simulink library "marine_gnc"  (Simulink 7.4)
settings: Solver=ode45  SolverMode=SingleTasking  StartTime=0.0  StopTime=10.0  RelTol=1e-3
undefined symbols (not defined in the file or in its folder): CN_data, CX_data, CY_data, D, G, K_supply, kt2ms, M, MA, magnitude, marine, Models, MRB, order, pathlength, RAO_Amp, RAO_Dir, RAO_Freq, RAO_Phase, RAO_Vel, RAO_yaw_back, RAO_yaw_quant, RAO_yaw_quantization_flag, rho_a, Semi, sub, T_supply, table, Tanker, vessel, Vessels
libraries: marine_gnc x64, simulink x39, cybersealib x1
(part 3 of 6)

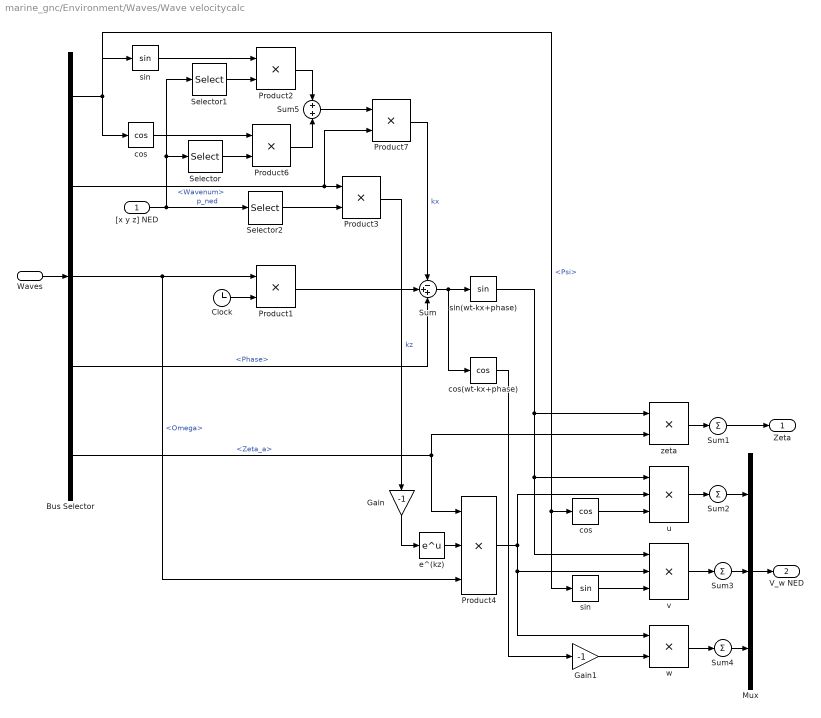
== system marine_gnc/Environment/Waves/Wave velocitycalc ==
  "[x y z] NED" : Inport  OutDataType=sfix(16)  OutScaling=2^0
  Waves : Inport  Port=2  OutDataType=sfix(16)  OutScaling=2^0
  Bus Selector : BusSelector  OutputSignals=Psi,Wavenum,Omega,Phase,Zeta_a
  Clock : Clock
      settings: Decimation=10
  Gain : Gain  Gain=-1  ParameterDataType=sfix(16)  ParameterScaling=2^0  OutDataType=sfix(16)  OutScaling=2^0  SaturateOnIntegerOverflow=on  OutDataTypeStr=Inherit: Same as input  ParamDataTypeStr=Inherit: Same as input
  Gain1 : Gain  Gain=-1  ParameterDataType=sfix(16)  ParameterScaling=2^0  OutDataType=sfix(16)  OutScaling=2^0  SaturateOnIntegerOverflow=on  OutDataTypeStr=Inherit: Same as input  ParamDataTypeStr=Inherit: Same as input
  Mux : Mux  Inputs=3
  Product{1..3,6..7} (5 alike) : Product  Inputs=**  OutDataType=sfix(16)  OutScaling=2^0  SaturateOnIntegerOverflow=on  OutDataTypeStr=Inherit: Same as first input
  Product4 : Product  Inputs=3  OutDataType=sfix(16)  OutScaling=2^0  SaturateOnIntegerOverflow=on  OutDataTypeStr=Inherit: Same as first input
  Selector : Selector  InputPortWidth=3  IndexOptions=Index vector (dialog)  Indices=1  OutputSizes=1
  Selector1 : Selector  InputPortWidth=3  IndexOptions=Index vector (dialog)  Indices=2  OutputSizes=1
  Selector2 : Selector  InputPortWidth=3  IndexOptions=Index vector (dialog)  Indices=3  OutputSizes=1
  Sum : Sum  Inputs=-++  OutDataType=sfix(16)  OutScaling=2^0  SaturateOnIntegerOverflow=on
  Sum{1..4} (4 alike) : Sum  Inputs=1  OutDataType=sfix(16)  OutScaling=2^0  SaturateOnIntegerOverflow=on
  Sum5 : Sum  OutDataType=sfix(16)  OutScaling=2^0  SaturateOnIntegerOverflow=on
  cos : Trigonometry  Operator=cos
  "cos " : Trigonometry  Operator=cos
  cos(wt-kx+phase) : Trigonometry  Operator=cos
  e^(kz) : Math  OutDataType=sfix(16)  OutScaling=2^0  SaturateOnIntegerOverflow=on
  sin : Trigonometry
  "sin " : Trigonometry
  sin(wt-kx+phase) : Trigonometry
  u : Product  Inputs=***  OutDataType=sfix(16)  OutScaling=2^0  SaturateOnIntegerOverflow=on  OutDataTypeStr=Inherit: Same as first input
  v : Product  Inputs=***  OutDataType=sfix(16)  OutScaling=2^0  SaturateOnIntegerOverflow=on  OutDataTypeStr=Inherit: Same as first input
  w : Product  Inputs=**  OutDataType=sfix(16)  OutScaling=2^0  SaturateOnIntegerOverflow=on  OutDataTypeStr=Inherit: Same as first input
  zeta : Product  Inputs=**  OutDataType=sfix(16)  OutScaling=2^0  SaturateOnIntegerOverflow=on  OutDataTypeStr=Inherit: Same as first input
  Zeta : Outport  OutDataType=sfix(16)  OutScaling=2^0
  V_w NED : Outport  Port=2  OutDataType=sfix(16)  OutScaling=2^0
  wires:
  Gain1/1 -> w/2
  "cos "/1 -> u/3
  "sin "/1 -> v/3
  Selector2/1 -> Product3/2
  "[x y z] NED"/1 -> Selector/1, Selector1/1, Selector2/1  "p_ned"
  Sum5/1 -> Product7/1
  Product6/1 -> Sum5/2
  Product2/1 -> Sum5/1
  sin/1 -> Product2/1
  Selector1/1 -> Product2/2
  cos/1 -> Product6/1
  Selector/1 -> Product6/2
  Bus Selector/2 -> Product3/1, Product7/2  "<Wavenum>"
  Gain/1 -> e^(kz)/1
  Bus Selector/5 -> Product4/1, zeta/2  "<Zeta_a>"
  Bus Selector/4 -> Sum/3  "<Phase>"
  Bus Selector/3 -> Product4/3, Product1/1  "<Omega>"
  Waves/1 -> Bus Selector/1
  cos(wt-kx+phase)/1 -> Gain1/1
  Product4/1 -> w/1, v/2, u/2
  e^(kz)/1 -> Product4/2
  Product7/1 -> Sum/1  "kx"
  zeta/1 -> Sum1/1
  sin(wt-kx+phase)/1 -> v/1, u/1, zeta/1
  Sum/1 -> cos(wt-kx+phase)/1, sin(wt-kx+phase)/1
  Product1/1 -> Sum/2
  Bus Selector/1 -> "cos "/1, "sin "/1, cos/1, sin/1  "<Psi>"
  Product3/1 -> Gain/1  "kz"
  Sum1/1 -> Zeta/1
  w/1 -> Sum4/1
  u/1 -> Sum2/1
  v/1 -> Sum3/1
  Sum2/1 -> Mux/1
  Sum3/1 -> Mux/2
  Sum4/1 -> Mux/3
  Mux/1 -> V_w NED/1
  Clock/1 -> Product1/2

== system marine_gnc/Environment/Waves/Waves ==
  Bus Creator : BusCreator  Inputs=5
  Omega : Constant  Value=Omega  OutDataType=sfix(16)  OutScaling=2^0
  Phase : Constant  Value=Phase  OutDataType=sfix(16)  OutScaling=2^0
  Psi : Constant  Value=Psi  OutDataType=sfix(16)  OutScaling=2^0
  Wavenum : Constant  Value=Wavenum  OutDataType=sfix(16)  OutScaling=2^0
  Zeta_a : Constant  Value=Zeta_a  OutDataType=sfix(16)  OutScaling=2^0
  "wave direction " : Constant  Value=psi_mean  OutDataType=sfix(16)  OutScaling=2^0
  Waves : Outport  OutDataType=sfix(16)  OutScaling=2^0
  wave direction : Outport  Port=2  OutDataType=sfix(16)  OutScaling=2^0
  wires:
  Phase/1 -> Bus Creator/5  "Phase"
  Psi/1 -> Bus Creator/2  "Psi"
  Omega/1 -> Bus Creator/1  "Omega"
  Bus Creator/1 -> Waves/1
  Zeta_a/1 -> Bus Creator/3  "Zeta_a"
  Wavenum/1 -> Bus Creator/4  "Wavenum"
  "wave direction "/1 -> wave direction/1

== system marine_gnc/Environment/Wind/Wind ==
  Gust : Constant  Value=Par_Wind_gust  OutDataType=sfix(16)  OutScaling=2^0
  Mean angle : Constant  Value=Par_Wind_angle  OutDataType=sfix(16)  OutScaling=2^0
  Mean velocity : Constant  Value=Par_Wind_V  OutDataType=sfix(16)  OutScaling=2^0
  Slowly-varying wind : Subsystem  mask(Slowly-varying wind){Par_Wind_sample_time=Par_Wind_sample_time, Par_Wind_speed_T=Par_Wind_speed_T, Par_Wind_angle_T=Par_Wind_angle_T, Par_Wind_speed_noise_pow=Par_Wind_speed_noise_pow, Par_Wind_angle_noise_pow=Par_Wind_angle_noise_pow, Par_Wind_speed_rand_max=Par_Wind_speed_rand_max, Par_Wind_angle_rand_max=Par_Wind_angle_rand_max, Par_Wind_speed_seed=Par_Wind_speed_seed, Par_Wind_angle_seed=Par_Wind_angle_seed}
      mask prompts: Par_Wind_sample_time "Wind sample time [s]"; Par_Wind_speed_T "Wind speed time constant [s]"; Par_Wind_angle_T "Wind angle time constant [s]"; Par_Wind_speed_noise_pow "Wind speed noise power"; Par_Wind_angle_noise_pow "Wind angle noise power"; Par_Wind_speed_rand_max "Wind speed saturation [m/s] (max random variation about mean)"; Par_Wind_angle_rand_max "Wind angle saturation [rad] (max random variation about mean)"; Par_Wind_speed_seed "Wind speed random seed"; Par_Wind_angle_seed "Wind angle random seed"
      mask help:
      | Generate slowly varying wind speed and direction based on random processes.
      |
      | stochastic = 0  gives constant mean wind speed and direction
      | stochastic = 1  gives stochastic mean wind speed and direction
      mask Help:
      | Generate slowly varying wind speed and direction based on random processes.<br>
      | <br>
      | stochastic = 0 gives constant mean wind direction and speed,<br>
      | stochastic = 1 gives stochastic mean wind direction and speed<br>
      | <br>
      | <p>The randomness of the mean speed and angle can be limited by two saturation
      | parameters, which define the maximum random deviation from the mean value.<br>
  Slowlyvar : Constant  Value=Par_Wind_slowlyvar  OutDataType=sfix(16)  OutScaling=2^0
  Sum : Sum  Inputs=++|  OutDataType=sfix(16)  OutScaling=2^0  SaturateOnIntegerOverflow=on
  Sum1 : Sum  Inputs=+++  OutDataType=sfix(16)  OutScaling=2^0  SaturateOnIntegerOverflow=on
  Wind gust : Subsystem  mask(Wind gust){Par_Wind_spectrum_type=Par_Wind_spectrum_type, Par_Wind_phase_seed=Par_Wind_phase_seed, Par_Wind_kappa_H=Par_Wind_kappa_H, Par_Wind_L=Par_Wind_L, Par_Wind_z=Par_Wind_z, Par_Wind_minfreq=Par_Wind_minfreq, Par_Wind_maxfreq=Par_Wind_maxfreq, Par_Wind_nfreq=Par_Wind_nfreq}
      mask prompts: Par_Wind_spectrum_type "Spectrum type"; Par_Wind_phase_seed "Wind gust phase seed"; Par_Wind_kappa_H "Sea surface drag coefficient for Harris wind spectrum (0.0026)"; Par_Wind_L "Scaling length for Harris wind spectrum (1800)"; Par_Wind_z "Height over water surface, for NORSOK spectrum"; Par_Wind_minfreq "Minimum frequency in gust [Hz] (1E-4)"; Par_Wind_maxfreq "Maximum frequency in gust [Hz] (0.1)"; Par_Wind_nfreq "Number of frequency components"
      mask help:
      | Calculate the wind gust according to one of two gust spectra:
      |
      | 1) Harris (based on measurements over land)
      | 2) NORSOK (based on measurements from the North Sea)
      |
      | The gust from the Harris spectrum is not influenced by the heigth over the sea surface, whereas the gust from the NORSOK spectrum is.
  angle : Outport  OutDataType=sfix(16)  OutScaling=2^0
  speed : Outport  Port=2  OutDataType=sfix(16)  OutScaling=2^0
  wires:
  Gust/1 -> Wind gust/Enable
  Slowlyvar/1 -> Slowly-varying wind/Enable
  Slowly-varying wind/1(angle) -> Sum/2
  Mean velocity/1 -> Wind gust/1(u10), Sum1/3
  Mean angle/1 -> Sum/1
  Sum/1 -> angle/1
  Wind gust/1(Gust) -> Sum1/2
  Slowly-varying wind/2(speed) -> Sum1/1
  Sum1/1 -> speed/1

== system marine_gnc/Examples/Applications/Autopilot - Kalman filter based wave filter using only compass ==
  Gain : Gain  ParameterDataType=sfix(16)  ParameterScaling=2^0  OutDataType=sfix(16)  OutScaling=2^0  SaturateOnIntegerOverflow=on  OutDataTypeStr=Inherit: Same as input  ParamDataTypeStr=Inherit: Same as input

== system marine_gnc/Examples/Applications/Autopilot - passive wave filter using compass/gyro ==
  Gain : Gain  ParameterDataType=sfix(16)  ParameterScaling=2^0  OutDataType=sfix(16)  OutScaling=2^0  SaturateOnIntegerOverflow=on  OutDataTypeStr=Inherit: Same as input  ParamDataTypeStr=Inherit: Same as input

== system marine_gnc/Examples/Applications/Autopilot - passive wave filter using only compass ==
  Gain : Gain  ParameterDataType=sfix(16)  ParameterScaling=2^0  OutDataType=sfix(16)  OutScaling=2^0  SaturateOnIntegerOverflow=on  OutDataTypeStr=Inherit: Same as input  ParamDataTypeStr=Inherit: Same as input

== system marine_gnc/Examples/Applications/DP system for CyberShipII ==
  Gain : Gain  ParameterDataType=sfix(16)  ParameterScaling=2^0  OutDataType=sfix(16)  OutScaling=2^0  SaturateOnIntegerOverflow=on  OutDataTypeStr=Inherit: Same as input  ParamDataTypeStr=Inherit: Same as input

== system marine_gnc/Examples/Applications/DP system for semi-submersible ==
  Gain : Gain  ParameterDataType=sfix(16)  ParameterScaling=2^0  OutDataType=sfix(16)  OutScaling=2^0  SaturateOnIntegerOverflow=on  OutDataTypeStr=Inherit: Same as input  ParamDataTypeStr=Inherit: Same as input

== system marine_gnc/Examples/Applications/Simulink interface for m-file vessel models ==
  Gain : Gain  ParameterDataType=sfix(16)  ParameterScaling=2^0  OutDataType=sfix(16)  OutScaling=2^0  SaturateOnIntegerOverflow=on  OutDataTypeStr=Inherit: Same as input  ParamDataTypeStr=Inherit: Same as input

== system marine_gnc/Examples/Applications/Thruster configuration demo for a supply vessel ==
  Gain : Gain  ParameterDataType=sfix(16)  ParameterScaling=2^0  OutDataType=sfix(16)  OutScaling=2^0  SaturateOnIntegerOverflow=on  OutDataTypeStr=Inherit: Same as input  ParamDataTypeStr=Inherit: Same as input

== system marine_gnc/Examples/Applications/Waves ==
  Gain : Gain  ParameterDataType=sfix(16)  ParameterScaling=2^0  OutDataType=sfix(16)  OutScaling=2^0  SaturateOnIntegerOverflow=on  OutDataTypeStr=Inherit: Same as input  ParamDataTypeStr=Inherit: Same as input

== system marine_gnc/Examples/Applications/Way-point guidance system ==
  Gain : Gain  ParameterDataType=sfix(16)  ParameterScaling=2^0  OutDataType=sfix(16)  OutScaling=2^0  SaturateOnIntegerOverflow=on  OutDataTypeStr=Inherit: Same as input  ParamDataTypeStr=Inherit: Same as input

== system marine_gnc/Examples/Applications/Zig-zag Test ==
  Gain : Gain  ParameterDataType=sfix(16)  ParameterScaling=2^0  OutDataType=sfix(16)  OutScaling=2^0  SaturateOnIntegerOverflow=on  OutDataTypeStr=Inherit: Same as input  ParamDataTypeStr=Inherit: Same as input

== system marine_gnc/Examples/Vessels/6 DOF supply vessel interface ==
  tau : Inport  OutDataType=sfix(16)  OutScaling=2^0
  3 to 6 DOF : marine_gnc/Models/ Kinetics /Support/3 to 6 DOF  SystemSampleTime=-1
  3 to 6 DOF1 : marine_gnc/Models/ Kinetics /Support/3 to 6 DOF  SystemSampleTime=-1
  6 to 3 DOF1 : Selector  InputPortWidth=6  IndexOptions=Index vector (dialog)  Indices=[1 2 6]  OutputSizes=1
  Supply vessel : marine_gnc/Examples/Vessels/Supply vessel  SystemSampleTime=-1  D=[5.0242e4 0 0; 0 2.7229e5 -4.3933e6; 0 -4.3933e6 4.1894e8]  Minv=inv( [5.3122e6 0 0; 0 8.2831e6 0; 0 0 3.7454e9] )
  eta : Outport  OutDataType=sfix(16)  OutScaling=2^0
  nu : Outport  Port=2  OutDataType=sfix(16)  OutScaling=2^0
  wires:
  3 to 6 DOF1/1 -> nu/1
  tau/1 -> 6 to 3 DOF1/1
  3 to 6 DOF/1 -> eta/1
  6 to 3 DOF1/1 -> Supply vessel/1
  Supply vessel/2 -> 3 to 6 DOF1/1
  Supply vessel/1 -> 3 to 6 DOF/1

== system marine_gnc/Examples/Vessels/CyberShipII ==
  note: etadot
  note: nu_dot
  note: nu
  tau : Inport  OutDataType=sfix(16)  OutScaling=2^0
  D : Gain  Gain=D  Multiplication=Matrix(K*u)  ParameterDataType=sfix(16)  ParameterScaling=2^0  OutDataType=sfix(16)  OutScaling=2^0  SaturateOnIntegerOverflow=on  OutDataTypeStr=Inherit: Same as input  ParamDataTypeStr=Inherit: Same as input
  Integrator1 : Integrator
  Integrator2 : Integrator
  Rotation matrix in yaw 1 : marine_gnc/Models/ Kinematics/Rotation matrix in yaw   SystemSampleTime=-1
  Sum3 : Sum  Inputs=+-  OutDataType=sfix(16)  OutScaling=2^0  SaturateOnIntegerOverflow=on  InputSameDT=on  OutDataTypeStr=Inherit: Same as first input
  inv(M) : Gain  Gain=inv(M)  Multiplication=Matrix(K*u)  ParameterDataType=sfix(16)  ParameterScaling=2^0  OutDataType=sfix(16)  OutScaling=2^0  SaturateOnIntegerOverflow=on  OutDataTypeStr=Inherit: Same as input  ParamDataTypeStr=Inherit: Same as input
  psi : Selector  InputPortWidth=3  IndexOptions=Index vector (dialog)  Indices=[3]  OutputSizes=1
  saturation : Subsystem
  eta : Outport  OutDataType=sfix(16)  OutScaling=2^0
  nu : Outport  Port=2  OutDataType=sfix(16)  OutScaling=2^0
  wires:
  saturation/1(sat_tau) -> Sum3/1
  psi/1 -> Rotation matrix in yaw 1/1
  Integrator1/1 -> psi/1, eta/1
  Rotation matrix in yaw 1/1 -> Integrator1/1
  inv(M)/1 -> Integrator2/1
  Sum3/1 -> inv(M)/1
  D/1 -> Sum3/2
  Integrator2/1 -> D/1, nu/1, Rotation matrix in yaw 1/2
  tau/1 -> saturation/1(tau)

== system marine_gnc/Examples/Vessels/Mariner class cargo ship  (2nd -order) ==
  rudder command : Inport  OutDataType=sfix(16)  OutScaling=2^0
  Integrator : Integrator
  Ship model : Subsystem
  Sum : Sum  Inputs=|+-  OutDataType=sfix(16)  OutScaling=2^0  SaturateOnIntegerOverflow=on  InputSameDT=on  OutDataTypeStr=Inherit: Same as first input
  rudder angle saturation : Saturate  UpperLimit=delta_max  LowerLimit=-delta_max
  rudder rate saturation : Saturate  UpperLimit=rate_max  LowerLimit=-rate_max
  heading angle : Outport  OutDataType=sfix(16)  OutScaling=2^0
  heading rate : Outport  Port=2  OutDataType=sfix(16)  OutScaling=2^0
  rudder angle : Outport  Port=3  OutDataType=sfix(16)  OutScaling=2^0
  wires:
  rudder command/1 -> rudder angle saturation/1
  Ship model/1(heading angle) -> heading angle/1
  Ship model/2(heading rate) -> heading rate/1
  Integrator/1 -> Sum/2, rudder angle/1, Ship model/1(rudder angle)
  rudder angle saturation/1 -> Sum/1
  Sum/1 -> rudder rate saturation/1
  rudder rate saturation/1 -> Integrator/1

== system marine_gnc/Examples/Vessels/Naval Vessel 4DOF (360ton) ==
  Tau (X,Y,K,N) : Inport  OutDataType=sfix(16)  OutScaling=2^0
  Initial Condition (u,v,p,r,phi,psi) : Constant  Value=ic  OutDataType=sfix(16)  OutScaling=2^0
  Selector : Selector  InputPortWidth=6  IndexOptions=Index vector (dialog)  Indices=[1 2 3 4]  OutputSizes=1
  Selector1 : Selector  InputPortWidth=6  IndexOptions=Index vector (dialog)  Indices=[5 6]  OutputSizes=1
  m-file interface : marine_gnc/Examples/Vessels/m-file interface  vessmodel=nv_nl_model  dimx_model=6
  Eta  (phi,psi) : Outport  OutDataType=sfix(16)  OutScaling=2^0
  Nu (u,v,p,r) : Outport  Port=2  OutDataType=sfix(16)  OutScaling=2^0
  wires:
  Tau (X,Y,K,N)/1 -> m-file interface/1
  Initial Condition (u,v,p,r,phi,psi)/1 -> m-file interface/2
  Selector/1 -> Nu (u,v,p,r)/1
  Selector1/1 -> Eta  (phi,psi)/1
  m-file interface/1 -> Selector1/1, Selector/1

== system marine_gnc/Examples/Vessels/Semi-sub ==
  tau : Inport  OutDataType=sfix(16)  OutScaling=2^0
  nu_c : Inport  Port=2  OutDataType=sfix(16)  OutScaling=2^0
  6 DOF Eqs. of motion : marine_gnc/Models/ Kinetics /6 DOF Eqs. of motion  CoriolisOnOff=on  nu0=[0 0 0 0 0 0]  eta0=[0 0 0 0 0 0]
  Constant : Constant  Value=MRB  OutDataType=sfix(16)  OutScaling=2^0
  "Constant " : Constant  Value=MA  OutDataType=sfix(16)  OutScaling=2^0
  D : Gain  Gain=D  Multiplication=Matrix(K*u)  ParameterDataType=sfix(16)  ParameterScaling=2^0  OutDataType=sfix(16)  OutScaling=2^0  SaturateOnIntegerOverflow=on  OutDataTypeStr=Inherit: Same as input  ParamDataTypeStr=Inherit: Same as input
  G : Gain  Gain=G  Multiplication=Matrix(K*u)  ParameterDataType=sfix(16)  ParameterScaling=2^0  OutDataType=sfix(16)  OutScaling=2^0  SaturateOnIntegerOverflow=on  OutDataTypeStr=Inherit: Same as input  ParamDataTypeStr=Inherit: Same as input
  Sum : Sum  Inputs=+--  OutDataType=sfix(16)  OutScaling=2^0  SaturateOnIntegerOverflow=on  InputSameDT=on  OutDataTypeStr=Inherit: Same as first input
  Sum1 : Sum  Inputs=-+|  OutDataType=sfix(16)  OutScaling=2^0  SaturateOnIntegerOverflow=on
  eta : Outport  OutDataType=sfix(16)  OutScaling=2^0  InitialOutput=0
  nu : Outport  Port=2  OutDataType=sfix(16)  OutScaling=2^0  InitialOutput=0
  wires:
  "Constant "/1 -> 6 DOF Eqs. of motion/2
  Sum/1 -> 6 DOF Eqs. of motion/3
  Sum1/1 -> D/1
  nu_c/1 -> Sum1/1, 6 DOF Eqs. of motion/4
  Constant/1 -> 6 DOF Eqs. of motion/1
  6 DOF Eqs. of motion/1 -> eta/1, G/1
  6 DOF Eqs. of motion/2 -> Sum1/2, nu/1
  G/1 -> Sum/2
  D/1 -> Sum/3
  tau/1 -> Sum/1

== system marine_gnc/Examples/Vessels/Supply vessel ==
  tau : Inport  OutDataType=sfix(16)  OutScaling=2^0
  D : Gain  Gain=D  Multiplication=Matrix(K*u)  ParameterDataType=sfix(16)  ParameterScaling=2^0  OutDataType=sfix(16)  OutScaling=2^0  SaturateOnIntegerOverflow=on  OutDataTypeStr=Inherit: Same as input  ParamDataTypeStr=Inherit: Same as input
  Integrator : Integrator
  Integrator1 : Integrator
  Minv : Gain  Gain=Minv  Multiplication=Matrix(K*u)  ParameterDataType=sfix(16)  ParameterScaling=2^0  OutDataType=sfix(16)  OutScaling=2^0  SaturateOnIntegerOverflow=on  OutDataTypeStr=Inherit: Same as input  ParamDataTypeStr=Inherit: Same as input
  "Rotation matrix in yaw " : marine_gnc/Models/ Kinematics/Rotation matrix in yaw 
  Sum : Sum  Inputs=+-  OutDataType=sfix(16)  OutScaling=2^0  SaturateOnIntegerOverflow=on  InputSameDT=on  OutDataTypeStr=Inherit: Same as first input
  yaw angle : Fcn  Expr=u(3)
  eta : Outport  OutDataType=sfix(16)  OutScaling=2^0  InitialOutput=0
  nu : Outport  Port=2  OutDataType=sfix(16)  OutScaling=2^0  InitialOutput=0
  wires:
  Integrator1/1 -> eta/1, yaw angle/1  "eta"
  Integrator/1 -> nu/1, "Rotation matrix in yaw "/2, D/1  "nu"
  yaw angle/1 -> "Rotation matrix in yaw "/1  "psi"
  "Rotation matrix in yaw "/1 -> Integrator1/1
  tau/1 -> Sum/1
  Minv/1 -> Integrator/1
  Sum/1 -> Minv/1
  D/1 -> Sum/2

== system marine_gnc/Examples/Vessels/Tanker (1st-order) ==
  rudder command : Inport  OutDataType=sfix(16)  OutScaling=2^0
  Integrator : Integrator
  Ship model : Subsystem
  Sum : Sum  Inputs=|+-  OutDataType=sfix(16)  OutScaling=2^0  SaturateOnIntegerOverflow=on  InputSameDT=on  OutDataTypeStr=Inherit: Same as first input
  rudder angle saturation : Saturate  UpperLimit=delta_max  LowerLimit=-delta_max
  rudder rate saturation : Saturate  UpperLimit=rate_max  LowerLimit=-rate_max
  heading angle : Outport  OutDataType=sfix(16)  OutScaling=2^0
  heading rate : Outport  Port=2  OutDataType=sfix(16)  OutScaling=2^0
  rudder angle : Outport  Port=3  OutDataType=sfix(16)  OutScaling=2^0
  wires:
  Ship model/2(heading rate) -> heading rate/1
  Ship model/1(heading angle) -> heading angle/1
  Integrator/1 -> Sum/2, Ship model/1(rudder angle), rudder angle/1
  rudder angle saturation/1 -> Sum/1
  Sum/1 -> rudder rate saturation/1
  rudder rate saturation/1 -> Integrator/1
  rudder command/1 -> rudder angle saturation/1

== system marine_gnc/Examples/Vessels/Tanker (2nd-order) ==
  rudder command : Inport  OutDataType=sfix(16)  OutScaling=2^0
  Integrator : Integrator
  Ship model : Subsystem
  Sum : Sum  Inputs=|+-  OutDataType=sfix(16)  OutScaling=2^0  SaturateOnIntegerOverflow=on  InputSameDT=on  OutDataTypeStr=Inherit: Same as first input
  rudder angle saturation : Saturate  UpperLimit=delta_max  LowerLimit=-delta_max
  rudder rate saturation : Saturate  UpperLimit=rate_max  LowerLimit=-rate_max
  heading angle : Outport  OutDataType=sfix(16)  OutScaling=2^0
  heading rate : Outport  Port=2  OutDataType=sfix(16)  OutScaling=2^0
  rudder angle : Outport  Port=3  OutDataType=sfix(16)  OutScaling=2^0
  wires:
  Ship model/1(heading angle) -> heading angle/1
  Ship model/2(heading rate) -> heading rate/1
  Integrator/1 -> Sum/2, Ship model/1(rudder angle), rudder angle/1
  rudder angle saturation/1 -> Sum/1
  Sum/1 -> rudder rate saturation/1
  rudder rate saturation/1 -> Integrator/1
  rudder command/1 -> rudder angle saturation/1

== system marine_gnc/Examples/Vessels/m-file examples ==
  Container ship: L = 175 m : Subsystem  mask(m-file vessel model interface){vessmodel='container', dimu_model=2, dimx_model=10}
      mask prompts: vessmodel "m-file vessel model"; dimu_model "dim u"; dimx_model "dim x"
      mask help:
      | Simulink interface to the GNC toolbox m-file vessel models, type:
      |
      |    >help vesselmodels
      |
      | in the Matlab command window. A Simulink demo file is found under examples (demomf.mdl).
      |
      | Inputs/outputs:
      |
      |    u   = control input vector of dimension dimu
      |    xo = initial state vector of dimension dimx
      |    x   = state vector of dimension dimx
      mask Help:
      | Simulink interface to the GNC toolbox m-file vessel models.
      | Type >help vesselmodels in the Matlab command window to see a list of the m-file vessel models. The dimension of the state and input vectors are found  by typing >help "m-file"
      mask Display:
      | disp('Integration of\n container.m\n\n...
      | x = [u v r x y psi p phi delta n]\n
      | u = [delta_c n_c]')
  Deep submergence rescue vehicle : Subsystem  mask(m-file vessel model interface){vessmodel='DSRV', dimu_model=1, dimx_model=5}
      mask prompts: vessmodel "m-file vessel model"; dimu_model "dim u"; dimx_model "dim x"
      mask help:
      | Simulink interface to the GNC toolbox m-file vessel models, type:
      |
      |    >help vesselmodels
      |
      | in the Matlab command window. A Simulink demo file is found under examples (demomf.mdl).
      |
      | Inputs/outputs:
      |
      |    u   = control input vector of dimension dimu
      |    xo = initial state vector of dimension dimx
      |    x   = state vector of dimension dimx
      mask Help:
      | Simulink interface to the GNC toolbox m-file vessel models.
      | Type >help vesselmodels in the Matlab command window to see a list of the m-file vessel models. The dimension of the state and input vectors are found  by typing >help "m-file"
      mask Display:
      | disp('Integration of\n DSRV.m\n\n...
      | x = [ w q x z theta ]\n
      | u = delta_s')
  Large tanker: L = 304 m : Subsystem  mask(m-file vessel model interface){vessmodel='tanker', dimu_model=3, dimx_model=8}
      mask prompts: vessmodel "m-file vessel model"; dimu_model "dim u"; dimx_model "dim x"
      mask help:
      | Simulink interface to the GNC toolbox m-file vessel models, type:
      |
      |    >help vesselmodels
      |
      | in the Matlab command window. A Simulink demo file is found under examples (demomf.mdl).
      |
      | Inputs/outputs:
      |
      |    u   = control input vector of dimension dimu
      |    xo = initial state vector of dimension dimx
      |    x   = state vector of dimension dimx
      mask Help:
      | Simulink interface to the GNC toolbox m-file vessel models.
      | Type >help vesselmodels in the Matlab command window to see a list of the m-file vessel models. The dimension of the state and input vectors are found  by typing >help "m-file"
      mask Display:
      | disp('Integration of\n tanker.m\n\n...
      | x = [u v r x y psi delta n]\n
      | u = [delta_c n_c h]')
  Mariner class vessel: L = 160 m : Subsystem  mask(m-file vessel model interface){vessmodel='mariner', dimu_model=1, dimx_model=7}
      mask prompts: vessmodel "m-file vessel model"; dimu_model "dim u"; dimx_model "dim x"
      mask help:
      | Simulink interface to the GNC toolbox m-file vessel models, type:
      |
      |    >help vesselmodels
      |
      | in the Matlab command window. A Simulink demo file is found under examples (demomf.mdl).
      |
      | Inputs/outputs:
      |
      |    u   = control input vector of dimension dimu
      |    xo = initial state vector of dimension dimx
      |    x   = state vector of dimension dimx
      mask Help:
      | Simulink interface to the GNC toolbox m-file vessel models.
      | Type >help vesselmodels in the Matlab command window to see a list of the m-file vessel models. The dimension of the state and input vectors are found  by typing >help "m-file"
      mask Display:
      | disp('Integration of\n mariner.m\n \n...
      | x = [ u v r x y psi delta] n\n...
      | u = delta_c')
  Naval Postgraduate School AUV : Subsystem  mask(m-file vessel model interface){vessmodel='npsauv', dimu_model=6, dimx_model=12}
      mask prompts: vessmodel "m-file vessel model"; dimu_model "dim u"; dimx_model "dim x"
      mask help:
      | Simulink interface to the GNC toolbox m-file vessel models, type:
      |
      |    >help vesselmodels
      |
      | in the Matlab command window. A Simulink demo file is found under examples (demomf.mdl).
      |
      | Inputs/outputs:
      |
      |    u   = control input vector of dimension dimu
      |    xo = initial state vector of dimension dimx
      |    x   = state vector of dimension dimx
      mask Help:
      | Simulink interface to the GNC toolbox m-file vessel models.
      | Type >help vesselmodels in the Matlab command window to see a list of the m-file vessel models. The dimension of the state and input vectors are found  by typing >help "m-file"
      mask Display:
      | disp('Integration of\n npsauv.m\n\n...
      | x = [u v w p q r x y z phi theta psi]\n...
      | u = [d_r d_s d_b d_bp d_bs n]')

== system marine_gnc/Examples/Vessels/m-file interface ==
  u : Inport  OutDataType=sfix(16)  OutScaling=2^0
  xo : Inport  Port=2  OutDataType=sfix(16)  OutScaling=2^0
  Integrator : Integrator  InitialConditionSource=external  InitialCondition=[1 1]  UpperSaturationLimit=10  LowerSaturationLimit=-10
  Mux1 : Mux  Inputs=2
  m-file : MATLABFcn  MATLABFcn=feval(vessmodel,u)  OutputDimensions=dimx_model  Output1D=off
  x : Outport  OutDataType=sfix(16)  OutScaling=2^0
  wires:
  m-file/1 -> Integrator/1
  Integrator/1 -> x/1, Mux1/1
  Mux1/1 -> m-file/1
  u/1 -> Mux1/2
  xo/1 -> Integrator/2

== system marine_gnc/Guidance/Way-point guidance block/Stop vessel ==
  theta : Inport  OutDataType=sfix(16)  OutScaling=2^0
  If endpoint1 : If  IfExpression=u1 > size(table,2)
  Merge : Merge
  Model Info : simulink/Model-Wide Utilities/Model Info  InitialBlockCM=None  BlockCM=None  Frame=on  DisplayStringWithTags=|  HorizontalTextAlignment=Center  LeftAlignmentValue=0.5  SourceBlockDiagram=marine_gnc  TagMaxNumber=20
      | Stop vessel
      | This subsystem performs an action when
      | the vessel reaches the last waypoint. The 
      | simultation is either stopped, or the desired 
      | speed is set to zero.
      | Author: Jorgen Corneliussen
      | Modified: %<ModifiedDate>
      | Version: %<ModelVersion>
  Reached endpoint : Subsystem  TreatAsAtomicUnit=on
  Still travelling : Subsystem  TreatAsAtomicUnit=on
  stopsignal : Outport  OutDataType=sfix(16)  OutScaling=2^0
  wires:
  Still travelling/1(one) -> Merge/2
  theta/1 -> If endpoint1/1
  If endpoint1/1 -> Reached endpoint/Action
  Reached endpoint/1(zero) -> Merge/1
  Merge/1 -> stopsignal/1
  If endpoint1/2 -> Still travelling/Action

== system marine_gnc/Guidance/Way-point guidance block/Thetacomputation ==
  theta : Inport  OutDataType=sfix(16)  OutScaling=2^0
  5th order algorithm : Subsystem  TreatAsAtomicUnit=on
  Constant1 : Constant  Value=method  OutDataType=sfix(16)  OutScaling=2^0
  Cubic splines : Subsystem  TreatAsAtomicUnit=on
  If endpoint1 : If  IfExpression=u1 == 1
  Model Info : simulink/Model-Wide Utilities/Model Info  InitialBlockCM=None  BlockCM=None  Frame=on  DisplayStringWithTags=|  HorizontalTextAlignment=Center  LeftAlignmentValue=0.5  SourceBlockDiagram=marine_gnc  TagMaxNumber=20
      | Thetacomputation
      | This subsystem returns a vector containing 
      | different orders of theta.
      | If cubic splines is used, the system returns:
      | [th^3 th^2 th 1]
      | If the 5th order polynomial is used, it returns:
      | [th^5 th^4 th^3 th^2 th 1]
      | Author: Jorgen Corneliussen
      | Modified: %<ModifiedDate>
      | Version: %<ModelVersion>
  Multiport Switch : MultiPortSwitch  Inputs=2  SaturateOnIntegerOverflow=on
  Selector : Selector  InputPortWidth=6  IndexOptions=Index vector (dialog)  Indices=[1:size(table,1)/8]  OutputSizes=1
  thetavector : Outport  OutDataType=sfix(16)  OutScaling=2^0
  wires:
  If endpoint1/1 -> Cubic splines/Action  "cubic"
  If endpoint1/2 -> 5th order algorithm/Action
  Constant1/1 -> If endpoint1/1, Multiport Switch/1
  theta/1 -> 5th order algorithm/1(theta), Cubic splines/1(theta)
  5th order algorithm/1(theta_vector) -> Multiport Switch/3
  Selector/1 -> thetavector/1
  Cubic splines/1(theta_vector) -> Multiport Switch/2
  Multiport Switch/1 -> Selector/1

== system marine_gnc/Guidance/Way-point guidance block/vs_calculations ==
  ud : Inport  OutDataType=sfix(16)  OutScaling=2^0
  ud_dot : Inport  Port=2  OutDataType=sfix(16)  OutScaling=2^0
  xd_theta : Inport  Port=3  OutDataType=sfix(16)  OutScaling=2^0
  yd_theta : Inport  Port=4  OutDataType=sfix(16)  OutScaling=2^0
  xd_theta_2 : Inport  Port=5  OutDataType=sfix(16)  OutScaling=2^0
  yd_theta_2 : Inport  Port=6  OutDataType=sfix(16)  OutScaling=2^0
  Model Info : simulink/Model-Wide Utilities/Model Info  InitialBlockCM=None  BlockCM=None  Frame=on  DisplayStringWithTags=|  HorizontalTextAlignment=Center  LeftAlignmentValue=0.5  SourceBlockDiagram=marine_gnc  TagMaxNumber=20
      | vs_calculations
      | This subsystem returns a vector containing 
      | the  speed assignment along the path.
      | The vector contains the desired speed, and 
      | the derivative of the desired speed with regards
      |  to theta and with regards to time.
      | Author: Jorgen Corneliussen
      | Modified: %<ModifiedDate>
      | Version: %<ModelVersion>
  vs_calc : Subsystem
  vs_t_calc : Subsystem
  vs_theta_calc : Subsystem
  vs : Outport  OutDataType=sfix(16)  OutScaling=2^0
  vs_theta : Outport  Port=2  OutDataType=sfix(16)  OutScaling=2^0
  vs_t : Outport  Port=3  OutDataType=sfix(16)  OutScaling=2^0
  wires:
  vs_calc/1(vs) -> vs/1  "vs"
  vs_theta_calc/1(vs_theta) -> vs_theta/1  "vs_theta"
  vs_t_calc/1(vs_t) -> vs_t/1  "vs_t"
  ud/1 -> vs_calc/1(ud), vs_theta_calc/5(ud)
  ud_dot/1 -> vs_t_calc/3(ud_dot)
  xd_theta/1 -> vs_calc/2(xd_theta), vs_theta_calc/1(xd_theta), vs_t_calc/1(xd_theta)
  yd_theta/1 -> vs_calc/3(yd_theta), vs_theta_calc/3(yd_theta), vs_t_calc/2(yd_theta)
  xd_theta_2/1 -> vs_theta_calc/2(xd_theta_2)
  yd_theta_2/1 -> vs_theta_calc/4(yd_theta_2)

== system marine_gnc/Models/ Kinematics/6 DOF transformation ==
  note: Theta
  note: v
  note: omega
  eta : Inport  OutDataType=sfix(16)  OutScaling=2^0
  nu : Inport  Port=2  OutDataType=sfix(16)  OutScaling=2^0
  Euler angles to rotation matrix1 : marine_gnc/Models/ Kinematics/Euler angles to rotation matrix  SystemSampleTime=-1
  Euler angles to attitude transformation matrix : marine_gnc/Models/ Kinematics/Euler angles to attitude transformation matrix  SystemSampleTime=-1
  Mux : Mux  Inputs=2
  Product : Product  Inputs=**  Multiplication=Matrix(*)  OutDataType=sfix(16)  OutScaling=2^0  SaturateOnIntegerOverflow=on  OutDataTypeStr=Inherit: Same as first input
  Product1 : Product  Inputs=**  Multiplication=Matrix(*)  OutDataType=sfix(16)  OutScaling=2^0  SaturateOnIntegerOverflow=on  OutDataTypeStr=Inherit: Same as first input
  Selector : Selector  InputPortWidth=6  IndexOptions=Index vector (dialog)  Indices=[4 5 6]  OutputSizes=1
  Selector1 : Selector  InputPortWidth=6  IndexOptions=Index vector (dialog)  Indices=[1 2 3]  OutputSizes=1
  Selector2 : Selector  InputPortWidth=6  IndexOptions=Index vector (dialog)  Indices=[4 5 6]  OutputSizes=1
  J(eta)*nu : Outport  OutDataType=sfix(16)  OutScaling=2^0
  wires:
  Selector/1 -> Euler angles to rotation matrix1/1, Euler angles to attitude transformation matrix/1
  eta/1 -> Selector/1
  Euler angles to rotation matrix1/1 -> Product/1
  nu/1 -> Selector1/1, Selector2/1
  Selector1/1 -> Product/2
  Selector2/1 -> Product1/2
  Euler angles to attitude transformation matrix/1 -> Product1/1
  Product/1 -> Mux/1
  Mux/1 -> J(eta)*nu/1
  Product1/1 -> Mux/2

== system marine_gnc/Models/ Kinematics/Euler angles to inverse rotation matrix ==
  theta : Inport  OutDataType=sfix(16)  OutScaling=2^0
  Mux2 : Mux  Inputs=2
  Mux3 : Mux  Inputs=9
  R11 : Fcn  Expr=u(5)*u(6)
  R12 : Fcn  Expr=u(5)*u(3)
  R13 : Fcn  Expr=-u(2)
  "R21 " : Fcn  Expr=-u(4)*u(3)+u(1)*u(2)*u(6)
  R22 : Fcn  Expr=u(4)*u(6)+u(1)*u(2)*u(3)
  R23 : Fcn  Expr=u(1)*u(5)
  "R31 " : Fcn  Expr=u(1)*u(3)+u(4)*u(2)*u(6)
  R32 : Fcn  Expr=-u(1)*u(6)+u(4)*u(2)*u(3)
  R33 : Fcn  Expr=u(4)*u(5)
  Reshape 9x1->3x3 : simulink/Math Operations/Reshape  OutputDimensionality=Customize  OutputDimensions=[3,3]
  cos(theta) : Trigonometry  Operator=cos
  sin(theta) : Trigonometry
  inv(R) : Outport  OutDataType=sfix(16)  OutScaling=2^0  InitialOutput=0
  wires:
  R33/1 -> Mux3/9
  R32/1 -> Mux3/6
  "R21 "/1 -> Mux3/2
  "R31 "/1 -> Mux3/3
  R12/1 -> Mux3/4
  R22/1 -> Mux3/5
  R13/1 -> Mux3/7
  R23/1 -> Mux3/8
  Mux2/1 -> R12/1, "R21 "/1, R11/1, "R31 "/1, R22/1, R23/1, R33/1, R13/1, R32/1
  theta/1 -> sin(theta)/1, cos(theta)/1
  cos(theta)/1 -> Mux2/2
  sin(theta)/1 -> Mux2/1
  Mux3/1 -> Reshape 9x1->3x3/1
  R11/1 -> Mux3/1
  Reshape 9x1->3x3/1 -> inv(R)/1

== system marine_gnc/Models/ Kinematics/Euler angles to rotation matrix ==
  theta : Inport  OutDataType=sfix(16)  OutScaling=2^0
  Mux : Mux  Inputs=2
  Mux2 : Mux  Inputs=9
  R11 : Fcn  Expr=u(6)*u(5)
  R12 : Fcn  Expr=u(6)*u(2)*u(1)-u(3)*u(4)
  R13 : Fcn  Expr=u(4)*u(2)*u(6)+u(3)*u(1)
  "R21 " : Fcn  Expr=u(3)*u(5)
  R22 : Fcn  Expr=u(3)*u(2)*u(1)+u(6)*u(4)
  R23 : Fcn  Expr=u(3)*u(2)*u(4)-u(6)*u(1)
  "R31 " : Fcn  Expr=-u(2)
  R32 : Fcn  Expr=u(5)*u(1)
  R33 : Fcn  Expr=u(5)*u(4)
  Reshape 9x1->3x3 : simulink/Math Operations/Reshape  OutputDimensionality=Customize  OutputDimensions=[3,3]
  cos(theta) : Trigonometry  Operator=cos
  sin(theta) : Trigonometry
  Rzyx : Outport  OutDataType=sfix(16)  OutScaling=2^0  InitialOutput=0
  wires:
  R11/1 -> Mux2/1
  Mux2/1 -> Reshape 9x1->3x3/1
  Reshape 9x1->3x3/1 -> Rzyx/1
  sin(theta)/1 -> Mux/1
  cos(theta)/1 -> Mux/2
  theta/1 -> sin(theta)/1, cos(theta)/1
  Mux/1 -> R32/1, R13/1, R33/1, R23/1, R22/1, "R31 "/1, R11/1, "R21 "/1, R12/1
  R23/1 -> Mux2/8
  R13/1 -> Mux2/7
  R22/1 -> Mux2/5
  R12/1 -> Mux2/4
  "R31 "/1 -> Mux2/3
  "R21 "/1 -> Mux2/2
  R32/1 -> Mux2/6
  R33/1 -> Mux2/9

== system marine_gnc/Models/ Kinematics/Euler angles to attitude transformation matrix ==
  theta : Inport  OutDataType=sfix(16)  OutScaling=2^0
  Constant : Constant  OutDataType=sfix(16)  OutScaling=2^0
  "Constant " : Constant  Value=0  OutDataType=sfix(16)  OutScaling=2^0
  Mux2 : Mux  Inputs=9
  Reshape 9x1->3x3 : simulink/Math Operations/Reshape  OutputDimensionality=Customize  OutputDimensions=[3,3]
  "T21 " : Fcn  Expr=sin(u(1))*tan(u(2))
  T22 : Fcn  Expr=cos(u(1))
  T23 : Fcn  Expr=sin(u(1))/cos(u(2))
  "T31 " : Fcn  Expr=cos(u(1))*tan(u(2))
  T32 : Fcn  Expr=-sin(u(1))
  T33 : Fcn  Expr=cos(u(1))/cos(u(2))
  T : Outport  OutDataType=sfix(16)  OutScaling=2^0  InitialOutput=0
  wires:
  Constant/1 -> Mux2/1
  Mux2/1 -> Reshape 9x1->3x3/1
  Reshape 9x1->3x3/1 -> T/1
  theta/1 -> T23/1, T33/1, T32/1, "T31 "/1, T22/1, "T21 "/1
  T23/1 -> Mux2/6
  T22/1 -> Mux2/5
  T33/1 -> Mux2/9
  "Constant "/1 -> Mux2/2, Mux2/3
  "T21 "/1 -> Mux2/4
  "T31 "/1 -> Mux2/7
  T32/1 -> Mux2/8

== system marine_gnc/Models/ Kinematics/Rotation matrix in yaw  ==
  psi : Inport  OutDataType=sfix(16)  OutScaling=2^0
  nu : Inport  Port=2  OutDataType=sfix(16)  OutScaling=2^0
  Fcn : Fcn  Expr=cos(u(1))*u(2)-sin(u(1))*u(3)
  Fcn1 : Fcn  Expr=sin(u(1))*u(2)+cos(u(1))*u(3)
  Fcn2 : Fcn  Expr=u(4)
  Mux : Mux  Inputs=2
  Mux1 : Mux  Inputs=3
  R*nu : Outport  OutDataType=sfix(16)  OutScaling=2^0
  wires:
  Mux/1 -> Fcn2/1, Fcn1/1, Fcn/1
  Fcn/1 -> Mux1/1  "x_dot"
  Fcn1/1 -> Mux1/2  "y_dot"
  Fcn2/1 -> Mux1/3  "psi_dot"
  Mux1/1 -> R*nu/1  "eta_dot"
  psi/1 -> Mux/1
  nu/1 -> Mux/2

== system marine_gnc/Models/ Kinematics/Transformation of generalized force ==
  tau : Inport  OutDataType=sfix(16)  OutScaling=2^0
  r_p : Inport  Port=2  OutDataType=sfix(16)  OutScaling=2^0
  Mux : Mux  Inputs=9
  Mux1 : Mux  Inputs=2
  Product : Product  Multiplication=Matrix(*)  OutDataType=sfix(16)  OutScaling=2^0  SaturateOnIntegerOverflow=on  OutDataTypeStr=Inherit: Same as first input
  Reshape 9x1 => 3x3 : simulink/Math Operations/Reshape  OutputDimensionality=Customize  OutputDimensions=[3,3]
  Selector1 : Selector  InputPortWidth=6  IndexOptions=Index vector (dialog)  Indices=[4 5 6]  OutputSizes=1
  Selector2 : Selector  InputPortWidth=6  IndexOptions=Index vector (dialog)  Indices=[1 2 3]  OutputSizes=1
  Sum : Sum  OutDataType=sfix(16)  OutScaling=2^0  SaturateOnIntegerOverflow=on
  h11 : Fcn  Expr=0
  h12 : Fcn  Expr=u(3)
  h13 : Fcn  Expr=-u(2)
  h21 : Fcn  Expr=-u(3)
  h22 : Fcn  Expr=0
  h23 : Fcn  Expr=u(1)
  h31 : Fcn  Expr=u(2)
  h32 : Fcn  Expr=-u(1)
  h33 : Fcn  Expr=0
  inv(H'(r_p))*tau : Outport  OutDataType=sfix(16)  OutScaling=2^0
  wires:
  tau/1 -> Selector1/1, Selector2/1
  Selector1/1 -> Sum/2  "m"
  Mux/1 -> Reshape 9x1 => 3x3/1
  Reshape 9x1 => 3x3/1 -> Product/1  "S'(r_12)"
  h11/1 -> Mux/1
  h21/1 -> Mux/2
  h31/1 -> Mux/3
  h12/1 -> Mux/4
  h22/1 -> Mux/5
  h32/1 -> Mux/6
  h13/1 -> Mux/7
  h23/1 -> Mux/8
  h33/1 -> Mux/9
  r_p/1 -> h11/1, h21/1, h31/1, h12/1, h22/1, h32/1, h13/1, h23/1, h33/1
  Mux1/1 -> inv(H'(r_p))*tau/1
  Selector2/1 -> Mux1/1, Product/2  "f"
  Sum/1 -> Mux1/2
  Product/1 -> Sum/1

== system marine_gnc/Models/ Kinematics/Transformation of generalized velocity ==
  note: S'(r_p)
  note: omega
  note: v
  nu : Inport  OutDataType=sfix(16)  OutScaling=2^0
  r_p : Inport  Port=2  OutDataType=sfix(16)  OutScaling=2^0
  Mux : Mux  Inputs=9
  Mux1 : Mux  Inputs=2
  Product : Product  Multiplication=Matrix(*)  OutDataType=sfix(16)  OutScaling=2^0  SaturateOnIntegerOverflow=on  OutDataTypeStr=Inherit: Same as first input
  Reshape 9x1 => 3x3 : simulink/Math Operations/Reshape  OutputDimensionality=Customize  OutputDimensions=[3,3]
  Selector1 : Selector  InputPortWidth=6  IndexOptions=Index vector (dialog)  Indices=[4 5 6]  OutputSizes=1
  Selector2 : Selector  InputPortWidth=6  IndexOptions=Index vector (dialog)  Indices=[1 2 3]  OutputSizes=1
  Sum : Sum  OutDataType=sfix(16)  OutScaling=2^0  SaturateOnIntegerOverflow=on
  h11 : Fcn  Expr=0
  h12 : Fcn  Expr=u(3)
  h13 : Fcn  Expr=-u(2)
  h21 : Fcn  Expr=-u(3)
  h22 : Fcn  Expr=0
  h23 : Fcn  Expr=u(1)
  h31 : Fcn  Expr=u(2)
  h32 : Fcn  Expr=-u(1)
  h33 : Fcn  Expr=0
  H(r_p)*nu : Outport  OutDataType=sfix(16)  OutScaling=2^0
  wires:
  Selector2/1 -> Sum/2
  Product/1 -> Sum/1
  Selector1/1 -> Product/2, Mux1/2
  Sum/1 -> Mux1/1
  Mux1/1 -> H(r_p)*nu/1
  r_p/1 -> h33/1, h23/1, h13/1, h32/1, h22/1, h12/1, h31/1, h21/1, h11/1
  h33/1 -> Mux/9
  h23/1 -> Mux/8
  h13/1 -> Mux/7
  h32/1 -> Mux/6
  h22/1 -> Mux/5
  h12/1 -> Mux/4
  h31/1 -> Mux/3
  h21/1 -> Mux/2
  h11/1 -> Mux/1
  Reshape 9x1 => 3x3/1 -> Product/1
  Mux/1 -> Reshape 9x1 => 3x3/1
  nu/1 -> Selector2/1, Selector1/1

== system marine_gnc/Models/ Kinematics/Transposed rotation  matrix in yaw ==
  psi : Inport  OutDataType=sfix(16)  OutScaling=2^0
  nu : Inport  Port=2  OutDataType=sfix(16)  OutScaling=2^0
  Mux : Mux  Inputs=2
  Mux1 : Mux  Inputs=3
  Row1 : Fcn  Expr=cos(u(1))*u(2)+sin(u(1))*u(3)
  Row2 : Fcn  Expr=-sin(u(1))*u(2)+cos(u(1))*u(3)
  Row3 : Fcn  Expr=u(4)
  Out1 : Outport  OutDataType=sfix(16)  OutScaling=2^0
  wires:
  nu/1 -> Mux/2
  psi/1 -> Mux/1
  Mux1/1 -> Out1/1
  Row3/1 -> Mux1/3
  Row2/1 -> Mux1/2
  Row1/1 -> Mux1/1
  Mux/1 -> Row1/1, Row2/1, Row3/1

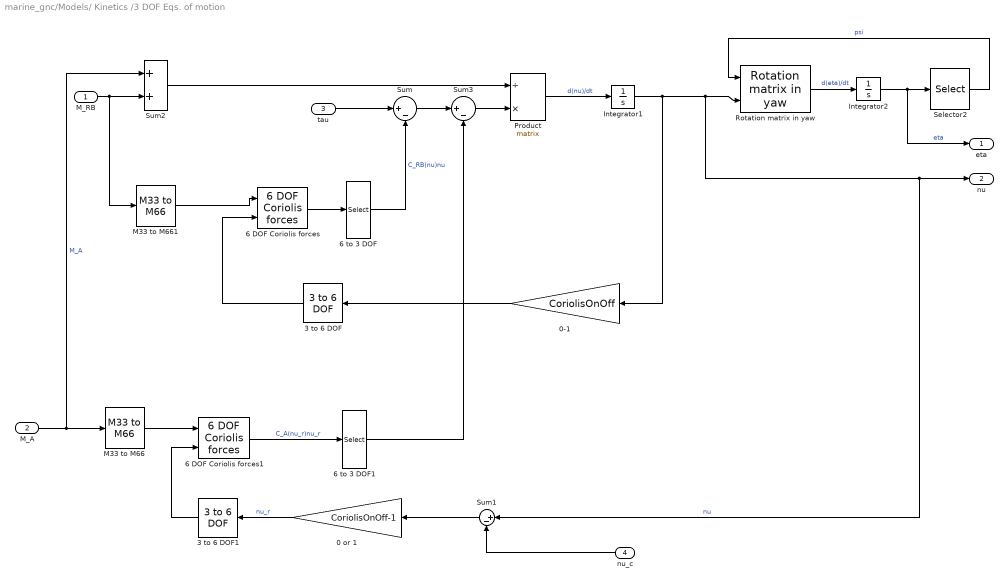
== system marine_gnc/Models/ Kinetics /3 DOF Eqs. of motion ==
  M_RB : Inport  OutDataType=sfix(16)  OutScaling=2^0
  M_A : Inport  Port=2  OutDataType=sfix(16)  OutScaling=2^0
  tau : Inport  Port=3  OutDataType=sfix(16)  OutScaling=2^0
  nu_c : Inport  Port=4  OutDataType=sfix(16)  OutScaling=2^0
  "0 or 1   " : Gain  Gain=CoriolisOnOff-1  ParameterDataType=sfix(16)  ParameterScaling=2^0  OutDataType=sfix(16)  OutScaling=2^0  SaturateOnIntegerOverflow=on  OutDataTypeStr=Inherit: Same as input  ParamDataTypeStr=Inherit: Same as input
  0-1 : Gain  Gain=CoriolisOnOff  ParameterDataType=sfix(16)  ParameterScaling=2^0  OutDataType=sfix(16)  OutScaling=2^0  SaturateOnIntegerOverflow=on  OutDataTypeStr=Inherit: Same as input  ParamDataTypeStr=Inherit: Same as input
  3 to 6 DOF : marine_gnc/Models/ Kinetics /Support/3 to 6 DOF
  3 to 6 DOF1 : marine_gnc/Models/ Kinetics /Support/3 to 6 DOF
  6 DOF Coriolis forces : marine_gnc/Models/ Kinetics /Support/6 DOF Coriolis forces
  6 DOF Coriolis forces1 : marine_gnc/Models/ Kinetics /Support/6 DOF Coriolis forces
  6 to 3 DOF : Selector  InputPortWidth=6  IndexOptions=Index vector (dialog)  Indices=[1 2 6]  OutputSizes=1
  6 to 3 DOF1 : Selector  InputPortWidth=6  IndexOptions=Index vector (dialog)  Indices=[1 2 6]  OutputSizes=1
  Integrator1 : Integrator  InitialCondition=nu0
  Integrator2 : Integrator  InitialCondition=eta0
  M33 to M66 : marine_gnc/Models/ Kinetics /Support/M33 to M66
  M33 to M661 : marine_gnc/Models/ Kinetics /Support/M33 to M66
  Product : Product  Inputs=/*  Multiplication=Matrix(*)  OutDataType=sfix(16)  OutScaling=2^0  SaturateOnIntegerOverflow=on  OutDataTypeStr=Inherit: Same as first input
  "Rotation matrix in yaw " : marine_gnc/Models/ Kinematics/Rotation matrix in yaw 
  Selector2 : Selector  InputPortWidth=3  IndexOptions=Index vector (dialog)  Indices=[3]  OutputSizes=1
  Sum : Sum  Inputs=|+-  OutDataType=sfix(16)  OutScaling=2^0  SaturateOnIntegerOverflow=on
  Sum1 : Sum  Inputs=|+-  OutDataType=sfix(16)  OutScaling=2^0  SaturateOnIntegerOverflow=on
  Sum2 : Sum  OutDataType=sfix(16)  OutScaling=2^0  SaturateOnIntegerOverflow=on
  Sum3 : Sum  Inputs=|+-  OutDataType=sfix(16)  OutScaling=2^0  SaturateOnIntegerOverflow=on
  eta : Outport  OutDataType=sfix(16)  OutScaling=2^0
  nu : Outport  Port=2  OutDataType=sfix(16)  OutScaling=2^0
  wires:
  6 to 3 DOF1/1 -> Sum3/2
  6 to 3 DOF/1 -> Sum/2  "C_RB(nu)nu"
  6 DOF Coriolis forces1/1 -> 6 to 3 DOF1/1  "C_A(nu_r)nu_r"
  Sum3/1 -> Product/2
  Sum/1 -> Sum3/1
  3 to 6 DOF1/1 -> 6 DOF Coriolis forces1/2
  M33 to M66/1 -> 6 DOF Coriolis forces1/1
  M_A/1 -> Sum2/1, M33 to M66/1  "M_A"
  nu_c/1 -> Sum1/2
  Sum1/1 -> "0 or 1   "/1
  "0 or 1   "/1 -> 3 to 6 DOF1/1  "nu_r"
  Sum2/1 -> Product/1
  M_RB/1 -> Sum2/2, M33 to M661/1
  Integrator1/1 -> 0-1/1, Sum1/1, nu/1, "Rotation matrix in yaw "/2  "nu"
  M33 to M661/1 -> 6 DOF Coriolis forces/1
  6 DOF Coriolis forces/1 -> 6 to 3 DOF/1
  3 to 6 DOF/1 -> 6 DOF Coriolis forces/2
  0-1/1 -> 3 to 6 DOF/1
  tau/1 -> Sum/1
  Selector2/1 -> "Rotation matrix in yaw "/1  "psi"
  Integrator2/1 -> eta/1, Selector2/1  "eta"
  "Rotation matrix in yaw "/1 -> Integrator2/1  "d(eta)/dt"
  Product/1 -> Integrator1/1  "d(nu)/dt"

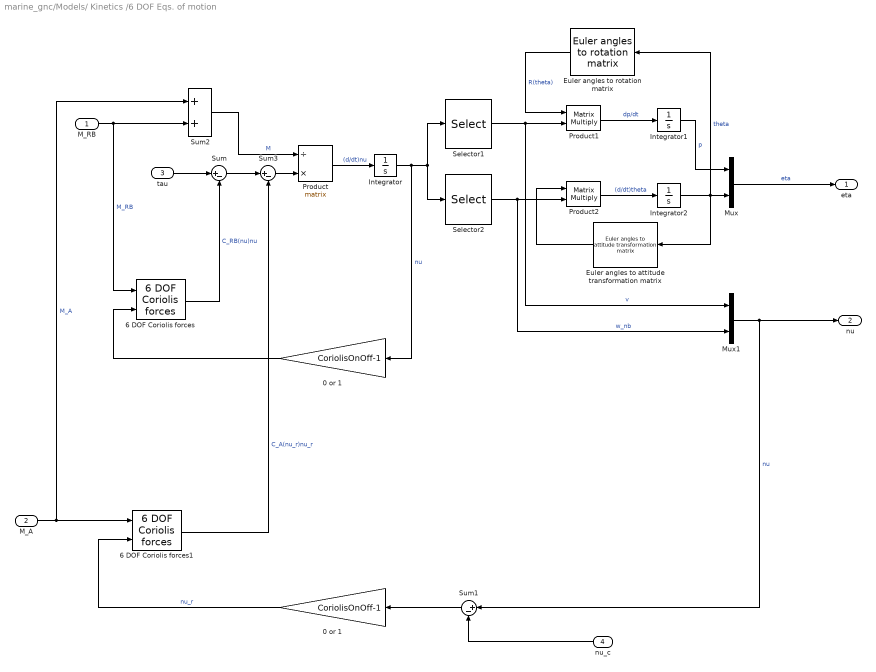
== system marine_gnc/Models/ Kinetics /6 DOF Eqs. of motion ==
  M_RB : Inport  OutDataType=sfix(16)  OutScaling=2^0
  M_A : Inport  Port=2  OutDataType=sfix(16)  OutScaling=2^0
  tau : Inport  Port=3  OutDataType=sfix(16)  OutScaling=2^0
  nu_c : Inport  Port=4  OutDataType=sfix(16)  OutScaling=2^0
  0 or 1 : Gain  Gain=CoriolisOnOff-1  ParameterDataType=sfix(16)  ParameterScaling=2^0  OutDataType=sfix(16)  OutScaling=2^0  SaturateOnIntegerOverflow=on  OutDataTypeStr=Inherit: Same as input  ParamDataTypeStr=Inherit: Same as input
  "0 or 1   " : Gain  Gain=CoriolisOnOff-1  ParameterDataType=sfix(16)  ParameterScaling=2^0  OutDataType=sfix(16)  OutScaling=2^0  SaturateOnIntegerOverflow=on  OutDataTypeStr=Inherit: Same as input  ParamDataTypeStr=Inherit: Same as input
  6 DOF Coriolis forces : marine_gnc/Models/ Kinetics /Support/6 DOF Coriolis forces
  6 DOF Coriolis forces1 : marine_gnc/Models/ Kinetics /Support/6 DOF Coriolis forces
  Euler angles to rotation matrix : marine_gnc/Models/ Kinematics/Euler angles to rotation matrix
  Euler angles to attitude transformation matrix : marine_gnc/Models/ Kinematics/Euler angles to attitude transformation matrix
  Integrator : Integrator  InitialCondition=nu0
  Integrator1 : Integrator  InitialCondition=eta0(1:3)
  Integrator2 : Integrator  InitialCondition=eta0(4:6)
  Mux : Mux  Inputs=2
  Mux1 : Mux  Inputs=2
  Product : Product  Inputs=/*  Multiplication=Matrix(*)  OutDataType=sfix(16)  OutScaling=2^0  SaturateOnIntegerOverflow=on  OutDataTypeStr=Inherit: Same as first input
  Product1 : Product  Inputs=**  Multiplication=Matrix(*)  OutDataType=sfix(16)  OutScaling=2^0  SaturateOnIntegerOverflow=on  OutDataTypeStr=Inherit: Same as first input
  Product2 : Product  Inputs=**  Multiplication=Matrix(*)  OutDataType=sfix(16)  OutScaling=2^0  SaturateOnIntegerOverflow=on  OutDataTypeStr=Inherit: Same as first input
  Selector1 : Selector  InputPortWidth=6  IndexOptions=Index vector (dialog)  Indices=[1 2 3]  OutputSizes=1
  Selector2 : Selector  InputPortWidth=6  IndexOptions=Index vector (dialog)  Indices=[4 5 6]  OutputSizes=1
  Sum : Sum  Inputs=|+-  OutDataType=sfix(16)  OutScaling=2^0  SaturateOnIntegerOverflow=on
  Sum1 : Sum  Inputs=|+-  OutDataType=sfix(16)  OutScaling=2^0  SaturateOnIntegerOverflow=on
  Sum2 : Sum  OutDataType=sfix(16)  OutScaling=2^0  SaturateOnIntegerOverflow=on
  Sum3 : Sum  Inputs=|+-  OutDataType=sfix(16)  OutScaling=2^0  SaturateOnIntegerOverflow=on
  eta : Outport  OutDataType=sfix(16)  OutScaling=2^0
  nu : Outport  Port=2  OutDataType=sfix(16)  OutScaling=2^0
  wires:
  nu_c/1 -> Sum1/2
  Sum1/1 -> "0 or 1   "/1
  "0 or 1   "/1 -> 6 DOF Coriolis forces1/2  "nu_r"
  6 DOF Coriolis forces1/1 -> Sum3/2  "C_A(nu_r)nu_r"
  Sum3/1 -> Product/2
  Sum/1 -> Sum3/1
  Sum2/1 -> Product/1  "M"
  M_A/1 -> Sum2/1, 6 DOF Coriolis forces1/1  "M_A"
  M_RB/1 -> Sum2/2, 6 DOF Coriolis forces/1  "M_RB"
  Product/1 -> Integrator/1  "(d/dt)nu"
  Integrator/1 -> Selector1/1, Selector2/1, 0 or 1/1  "nu"
  Selector1/1 -> Product1/2, Mux1/1  "v"
  Selector2/1 -> Mux1/2, Product2/2  "w_nb"
  Product1/1 -> Integrator1/1  "dp/dt"
  Euler angles to rotation matrix/1 -> Product1/1  "R(theta)"
  Product2/1 -> Integrator2/1  "(d/dt)theta"
  Integrator2/1 -> Mux/2, Euler angles to rotation matrix/1, Euler angles to attitude transformation matrix/1  "theta"
  Integrator1/1 -> Mux/1  "p"
  Mux/1 -> eta/1  "eta"
  Mux1/1 -> Sum1/1, nu/1  "nu"
  Euler angles to attitude transformation matrix/1 -> Product2/1
  tau/1 -> Sum/1
  6 DOF Coriolis forces/1 -> Sum/2  "C_RB(nu)nu"
  0 or 1/1 -> 6 DOF Coriolis forces/2

== system marine_gnc/Models/ Kinetics /Support ==
  3 to 6 DOF : Subsystem
      mask Display: disp('modes,\n 1,2,6, to\n 6 DOF')
  4 to 6 DOF : Subsystem
      mask Display: disp('modes,\n 1,2,4,6, to\n 6 DOF')
  6 DOF Coriolis forces : Subsystem
  6 to 3 DOF : Selector  InputPortWidth=6  IndexOptions=Index vector (dialog)  Indices=[1 2 6]  OutputSizes=1
  6 to 4 DOF : Selector  InputPortWidth=6  IndexOptions=Index vector (dialog)  Indices=[1 2 4 6]  OutputSizes=1
  M33 to M66 : Subsystem
      mask Display: disp('add zeros')
  M44 to M66 : Subsystem
      mask Display: disp('add zeros')
  M66 to M33 : Selector  NumberOfDimensions=2  InputPortWidth=3  IndexOptions=Index vector (dialog),Index vector (dialog)  Indices=[1 2 6],[1 2 6]  OutputSizes=1
  M66 to M44 : Selector  NumberOfDimensions=2  InputPortWidth=3  IndexOptions=Index vector (dialog),Index vector (dialog)  Indices=[1 2 4 6],[1 2 4 6]  OutputSizes=1

== system marine_gnc/Models/Control Surfaces/Fin/Rudder Machinery ==
  Angle Comm : Inport  OutDataType=sfix(16)  OutScaling=2^0
  Gain : Gain  Gain=1/tc  ParameterDataType=sfix(16)  ParameterScaling=2^0  OutDataType=sfix(16)  OutScaling=2^0  SaturateOnIntegerOverflow=on  OutDataTypeStr=Inherit: Same as input  ParamDataTypeStr=Inherit: Same as input
  Integrator : Integrator
  Saturation : Saturate  UpperLimit=Dvmax  LowerLimit=-Dvmax
  Saturation1 : Saturate  UpperLimit=Dmax  LowerLimit=-Dmax
  Sum : Sum  Inputs=|+-  OutDataType=sfix(16)  OutScaling=2^0  SaturateOnIntegerOverflow=on  InputSameDT=on  OutDataTypeStr=Inherit: Same as first input
  "Actual Ang. " : Outport  OutDataType=sfix(16)  OutScaling=2^0
  wires:
  Angle Comm/1 -> Saturation1/1
  Saturation/1 -> Integrator/1
  Saturation1/1 -> Sum/1
  Integrator/1 -> "Actual Ang. "/1, Sum/2
  Sum/1 -> Gain/1
  Gain/1 -> Saturation/1
